simulink model "repetitive_control"  (R2023b)
settings: Solver=FixedStepAuto  StartTime=0.0  StopTime=20  FixedStep=0.0025  RelTol=1e-3
libraries: dspsrcs4 x1
settings Model: Creator=Administrator  LastModifiedBy=Administrator

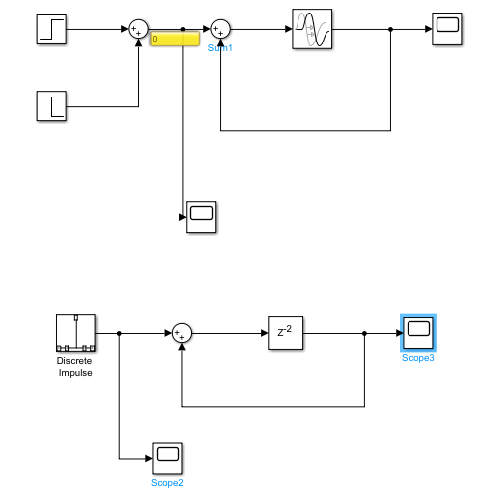
[thumbnail: Simulink's stored preview of the top-level diagram]
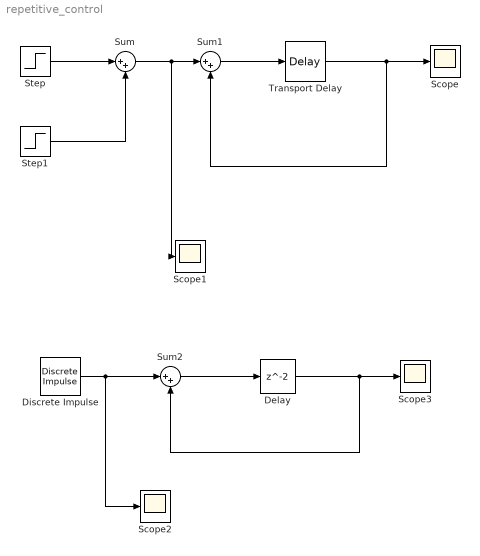
== system repetitive_control ==
  Delay : Delay
  Discrete Impulse : dspsrcs4/Discrete  Impulse  Delay=0  SampleTime=1  FrameSample=1  OutputFrames=off  dataType=double  isSigned=on  wordLen=16  udDataType=sfix(16)  fracBitsMode=Best precision  numFracBits=15  OutDataTypeStr=double  LastOutDataTypeStr=double
  Scope{,1..3} (4 alike) : Scope
  Step : Step  SampleTime=0
  Step1 : Step  Time=2  After=-1  SampleTime=0
  Sum : Sum  Inputs=|++
  Sum1 : Sum  Inputs=|++
  Sum2 : Sum  Inputs=|++
  Transport Delay : TransportDelay  DelayTime=2
  wires:
  Step/1 -> Sum/1
  Step1/1 -> Sum/2
  Sum/1 -> Scope1/1, Sum1/1
  Sum1/1 -> Transport Delay/1
  Transport Delay/1 -> Sum1/2, Scope/1
  Discrete Impulse/1 -> Sum2/1, Scope2/1
  Sum2/1 -> Delay/1
  Delay/1 -> Scope3/1, Sum2/2
